simulink model "Khaldoun_Caracteristiques_PV"  (Simulink 8.5)
settings: Solver=ode45  StartTime=0.0  StopTime=0.005  RelTol=1e-3
undefined symbols (not defined in the file or in its folder): Ts_Power
libraries: powerlib x9, simulink x1
settings Model: Creator=Khaled  LastModifiedBy=ironi
settings DebuggingCC: SolverPrmCheckMsg=warning  FcnCallInpInsideContextMsg=EnableAllAsWarning
settings GRTTargetCC: CombineOutputUpdateFcns=on  GRTInterface=off

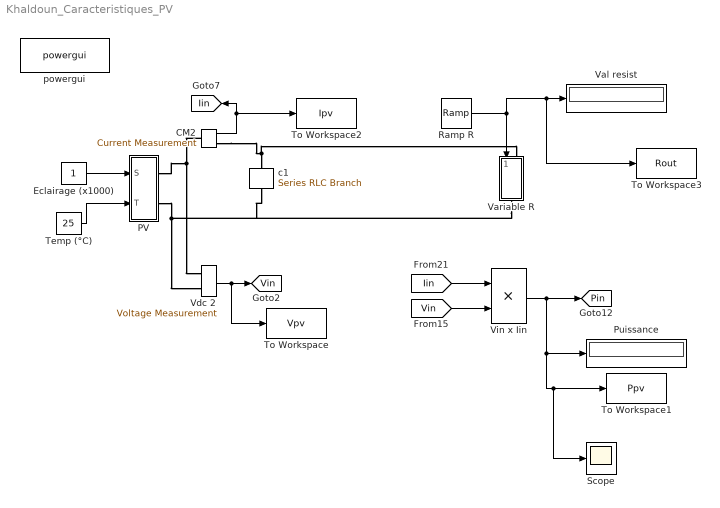
== system Khaldoun_Caracteristiques_PV ==
  CM2 : powerlib/Measurements/Current Measurement  Tag=PoWeRsYsTeMmEaSuReMeNt  PhasorSimulation=off  OutputType=Magnitude  PSBequivalent=0
  Eclairage (x1000) : Constant
  "PV " : Subsystem
  Puissance : Display
      settings: Format=bank  Decimation=100
  Ramp R : simulink/Sources/Ramp  slope=200000  start=0  X0=2
  Scope : Scope
  Temp (°C) : Constant  Value=25
  To Workspace : ToWorkspace  VariableName=Vpv  SampleTime=-1
  To Workspace1 : ToWorkspace  VariableName=Ppv  SampleTime=-1
  To Workspace2 : ToWorkspace  VariableName=Ipv  SampleTime=-1
  To Workspace3 : ToWorkspace  VariableName=Rout  SampleTime=-1
  Val resist : Display
      settings: Format=bank  Decimation=100
  Variable R : Subsystem
  Vdc 2 : powerlib/Measurements/Voltage Measurement  Tag=PoWeRsYsTeMmEaSuReMeNt  PhasorSimulation=off  OutputType=Magnitude  PSBequivalent=0
  Vin x Iin : Product  RndMeth=Zero
  c1 : powerlib/Elements/Series RLC Branch  LConnTagsString=__new0  RConnTagsString=__new0  BranchType=C  Resistance=0.01  Inductance=1.0  SetiL0=off  InitialCurrent=0  Capacitance=3e-6  Setx0=on  InitialVoltage=0  Measurements=None
  powergui : powerlib/powergui  Priority=1  SimulationMode=Continuous  SolverType=Tustin  SampleTime=Ts_Power  frequency=60  SPID=off  DisableSnubberDevices=off  DisableRonSwitches=off  DisableVfSwitches=off  SwTol=0  DisplayEquations=off  Interpol=off  methode=off  Ts=0  FunctionMessages=off  echomessages=off  HookPort=off  EnableUseOfTLC=off  x0status=blocks  frequencyindice=0  Pbase=100e6  ErrMax=1e-4  Iterations=50  UnitsV=kV  UnitsW=MW  buscounter=0  RestoreLinks=warning  ResistiveCurrentMeasurement=off  Frange=[0:2:500]  Ylog=off  Xlog=on  ShowGrid=off  save=off  variable=ZData  structure=0  ZoomFFT=on  StartTime=0.0  cycles=1  DisplayStyle=1  fundamental=60  FreqAxis=off  MaxFrequency=1000  frequencyindicesteady=1  RmsSteady=1  display=off
  tag scope: Iin=global, Pin=global, Vin=global
  wires:
  [Iin] -> Vin x Iin/1
  [Vin] -> Vin x Iin/2
  Vin x Iin/1 -> [Pin], Puissance/1, Scope/1, To Workspace1/1
  CM2/1 -> [Iin], To Workspace2/1
  Vdc 2/1 -> [Vin], To Workspace/1
  Ramp R/1 -> Variable R/1(Var R), To Workspace3/1, Val resist/1
  Eclairage (x1000)/1 -> "PV "/1(S)
  Temp (°C)/1 -> "PV "/2(T)
  connections:
  "PV "/RConn1 -- Vdc 2/LConn1 -- CM2/LConn1
  "PV "/RConn2 -- Variable R/RConn1 -- c1/RConn1 -- Vdc 2/LConn2
  c1/LConn1 -- CM2/RConn1 -- Variable R/LConn1

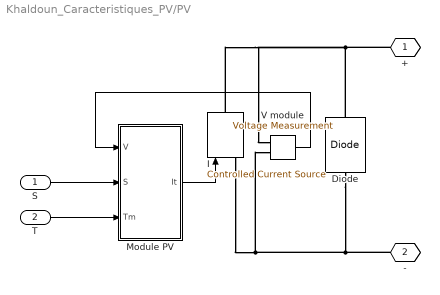
== system Khaldoun_Caracteristiques_PV/PV  ==
  S : Inport
  T : Inport  Port=2
  Diode : powerlib/Power Electronics/Diode  Ron=0.001  Lon=0  Vf=0  IC=0  UseSnubber=off  Rs=500  Cs=250e-9  Measurements=off
  I : powerlib/Electrical Sources/Controlled Current Source  Initialize=on  Source_Type=AC  Amplitude=0  Phase=0  Frequency=0  Measurements=None
  Module PV : MATLAB Function  TreatAsAtomicUnit=on
  V module : powerlib/Measurements/Voltage Measurement  PhasorSimulation=off  OutputType=Complex  PSBequivalent=0
      link override source: GotoTag=tp967389f0_fd12_437c_b6ba_935a91dc4f07
  + : PMIOPort  Tag=PMCPort  Port=1  Side=Right
  - : PMIOPort  Tag=PMCPort  Port=2  Side=Right
  wires:
  Module PV/1(It) -> I/1
  V module/1 -> Module PV/1(V)
  S/1 -> Module PV/2(S)
  T/1 -> Module PV/3(Tm)
  connections:
  -/RConn1 -- I/LConn1 -- V module/LConn2 -- Diode/LConn1
  +/RConn1 -- I/RConn1 -- V module/LConn1 -- Diode/RConn1

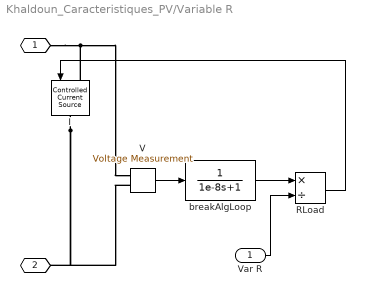
== system Khaldoun_Caracteristiques_PV/Variable R ==
  Var R : Inport
  I : powerlib/Electrical Sources/Controlled Current Source  Initialize=on  Source_Type=DC  Amplitude=0  Phase=0  Frequency=0  Measurements=None
  RLoad : Product  Inputs=*/  RndMeth=Zero
  V : powerlib/Measurements/Voltage Measurement  PhasorSimulation=off  OutputType=Complex  PSBequivalent=0
  breakAlgLoop : TransferFcn  Denominator=[1e-8 1]
  " " : PMIOPort  Port=1  Side=Left
  "   " : PMIOPort  Port=2  Side=Right
  wires:
  Var R/1 -> RLoad/2
  breakAlgLoop/1 -> RLoad/1
  V/1 -> breakAlgLoop/1
  RLoad/1 -> I/1
  connections:
  I/LConn1 -- V/LConn1 -- " "/RConn1
  I/RConn1 -- V/LConn2 -- "   "/RConn1

== matlab function PV /Module PV ==
  data: V input double; It output double; S input double; Tm input double
function It=ISolaire(V,S,Tm) 
% Sortie:      It = courant du module (A)
% Entrees:     V = tension du module (V)
%              S = irradiance ; avec 1S => 1000 (W/m^2)
%              Tm = temperature du module (°C)
%----------------------------------------------------------------------
k = 1.381e-23;      % cste de Boltzmann  
q = 1.602e-19;      % charge electron 
% A = 1.81;           % facteur de idealité de la diode (1<A<2)
A = 1.3;           % facteur de idealité de la diode (1<A<2)
Eg = 1.16;          % energie de bandgap du semi-conducteur (eV)
% Ns = 72;            % cellules en =
Ns = 1;            % cellules en =
Np = 1;               % cellules en //
ki=1.96e-3;         % Coefficient de température de court-circuit(A/°K)
% Rs =2.48e-3;        % résistance serie(Ohm)
Rs =0.221;        % résistance serie(Ohm)
% Rp = 8.7;           % résistance parallele(Ohm)
Rp = 50;           % résistance parallele(Ohm)
Tr =298.5;          % temperature de reference en (K)
% I0_r = 1.13e-6;     % courant inverse de référence
I0_r = 9.825e-8;     % courant inverse de référence
% Ir_ph = 5.61;       % (A) courant de c-c de référence
Ir_ph = 0.015;       % (A) courant de c-c de référence
T = 273 + Tm;       % Temp du module en (K)

Iph= (Ir_ph + ki*(T-Tr))*(S); %courant genere

I0=I0_r*((T/Tr)^(3)) *exp((q*Eg/(A*k))*(1/Tr - 1/T)); % courant inverse

Vt=(A*k*T)/q; % tension thermique 

%I= Iph- I0*(exp((V/Ns + I*Rs)/Vt) -1) - (((V/ns + I*Rs)/Rp))
% f(I) = Iph - I - I0*(exp((V/Ns + I*Rs)/Vt) -1) - (((V/ns + I*Rs)/Rp)) = 0 
% Solution pour passer la boucle algébrique avec la methode de Newton: I2 = I1 - f(I1)/f'(I1) 
% I=zeros(size(Vc)); % Initialiser I avec zeros   
I=zeros(size(V)); % Initialiser I avec zeros   

for j=1:5; 
    I = I - (Iph - I - I0 .* ( exp((V/Ns + I .* Rs) ./ Vt) -1) -((V/Ns + I .* Rs)/Rp))... 
        ./ ((-1 - I0 * (Rs ./ Vt) .* exp((V/Ns + I .* Rs) ./ Vt)) -Rs/Rp); 
end
It=I*Np;  % courant totale du module

end
